simulink model "Control_car_position"  (R2022a)
settings: Solver=VariableStepAuto  StartTime=0.0  StopTime=100  RelTol=1e-3
libraries: slpidlib x5, simulink_extras x3
settings Model: Creator=jvlsq  LastModifiedBy=jvlsq
settings SolverCC: ZeroCrossAlgorithm=Adaptive
settings DebuggingCC: IgnoredZcDiagnostic=none

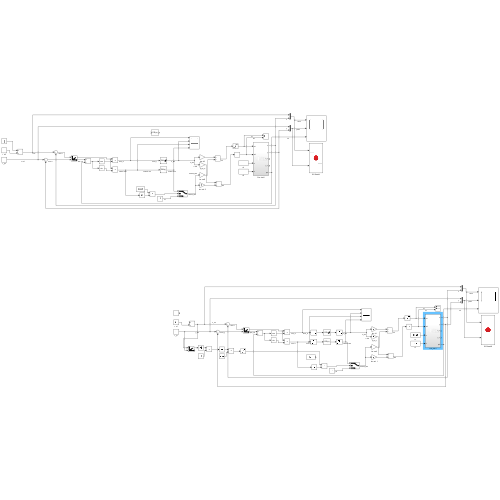
[thumbnail: Simulink's stored preview of the top-level diagram]
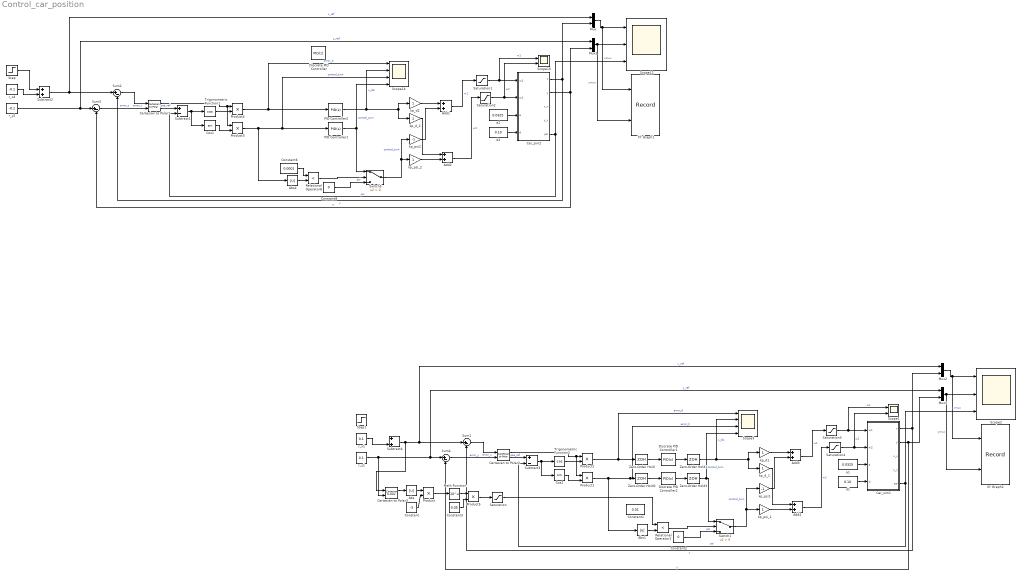
== system Control_car_position ==
  Abs : Abs  SaturateOnIntegerOverflow=off
  Abs1 : Abs  SaturateOnIntegerOverflow=off
  Abs4 : Abs  SaturateOnIntegerOverflow=off
  Add{1..4} (4 alike) : Sum
  Car_sim1 : Subsystem
  Car_sim2 : Subsystem
  Cartesian to Polar1 : simulink_extras/Transformations/Cartesian to Polar
  Cartesian to Polar2 : simulink_extras/Transformations/Cartesian to Polar
  Cartesian to Polar3 : simulink_extras/Transformations/Cartesian to Polar
  Constant : Constant  Value=-3
  Constant1 : Constant  Value=0.01
  Constant2 : Constant  Value=0
  Constant3 : Constant  Value=0.05
  Constant6 : Constant  Value=0.0001
  Constant8 : Constant  Value=0
  Cos1 : Trigonometry
  Cos2 : Trigonometry
  Discrete PID Controller : slpidlib/PID Controller  Controller=PID  Form=Parallel  TimeDomain=Discrete-time  UseExternalTs=off  SampleTime=-1  IntegratorMethod=Forward Euler  FilterMethod=Forward Euler  ControllerParametersSource=internal  P=1  I=1  UseKiTs=off  D=0  N=100  UseFilter=on  TunerSelectOption=Transfer Function Based (PID Tuner App)  InitialConditionSource=internal  InitialConditionForIntegrator=0  InitialConditionForFilter=0  DifferentiatorICPrevScaledInput=0  ExternalReset=none  TrackingMode=off  Kt=1  LimitOutput=off  SatLimitsSource=internal  UpperSaturationLimit=inf  LowerSaturationLimit=-inf  LinearizeAsGain=off  AntiWindupMode=none  Kb=1  POutMin=[]  POutMax=[]  IOutMin=[]  IOutMax=[]  DOutMin=[]  DOutMax=[]  NOutMin=[]  NOutMax=[]  SumOutMin=[]  SumOutMax=[]  SaturationOutMin=[]  SaturationOutMax=[]  PParamMin=[]  PParamMax=[]  IParamMin=[]  IParamMax=[]  DParamMin=[]  DParamMax=[]  NParamMin=[]  NParamMax=[]  KbParamMin=[]  KbParamMax=[]  KtParamMin=[]  KtParamMax=[]  KbOutMin=[]  KbOutMax=[]  KtOutMin=[]  KtOutMax=[]  IntegratorOutMin=[]  IntegratorOutMax=[]  FilterOutMin=[]  FilterOutMax=[]  SumI1OutMin=[]  SumI1OutMax=[]  SumI2OutMin=[]  SumI2OutMax=[]  SumI3OutMin=[]  SumI3OutMax=[]  SumI4OutMin=[]  SumI4OutMax=[]  SumDOutMin=[]  SumDOutMax=[]  DifferentiatorOutMin=[]  DifferentiatorOutMax=[]  FilterDiffOutCoefMin=[]  FilterDiffOutCoefMax=[]  ReciprocalOutMin=[]  ReciprocalOutMax=[]  SumDenOutMin=[]  SumDenOutMax=[]  SumNumOutMin=[]  SumNumOutMax=[]  DivideOutMin=[]  DivideOutMax=[]  UdiffTsProdOutMin=[]  UdiffTsProdOutMax=[]  NTsProdOutMin=[]  NTsProdOutMax=[]  UintegralTsProdOutMin=[]  UintegralTsProdOutMax=[]  UngainTsProdOutMin=[]  UngainTsProdOutMax=[]  IntegratorContinuousStateAttributes=''  IntegratorStateMustResolveToSignalObject=off  IntegratorRTWStateStorageClass=Auto  FilterContinuousStateAttributes=''  FilterStateMustResolveToSignalObject=off  FilterRTWStateStorageClass=Auto  ParallelPVariant=InternalParameters  IdealPVariant=Disabled  IVariant=InternalParameters  DVariant=InternalParameters  IntegratorVariant=Discrete  SatVariant=Disabled  AWVariant=Passthrough  PCopyVariant=Disabled  TRVariant=Disabled  FdbkBlocksVariant=Forward  IdealPFdbkVariant=Disabled  SatFdbkVariant=Disabled  DerivativeFilterVariant=ForwardEulerFilter  NVariant=InternalParameters  NCopyVariant=Disabled  FilterICVariant=InternalICsFilter  IntegratorICVariant=InternalICs  ExternalResetVariant=Disabled  TRSumVariant=Passthrough  SumFdbkVariant=Disabled  SumVariant=Sum_PID  TsampFilterVariant=InternalTs  TsampNgainVariant=Passthrough  TsampIntegralVariant=Passthrough  ExternalSaturationOutDataTypeStr=Inherit: Same as second input  aMode=0
  Discrete PID Controller1 : slpidlib/PID Controller  Controller=PID  Form=Parallel  TimeDomain=Discrete-time  UseExternalTs=off  SampleTime=-1  IntegratorMethod=Forward Euler  FilterMethod=Forward Euler  ControllerParametersSource=internal  P=30  I=1  UseKiTs=off  D=0  N=100  UseFilter=on  TunerSelectOption=Transfer Function Based (PID Tuner App)  InitialConditionSource=internal  InitialConditionForIntegrator=0  InitialConditionForFilter=0  DifferentiatorICPrevScaledInput=0  ExternalReset=none  TrackingMode=off  Kt=1  LimitOutput=on  SatLimitsSource=internal  UpperSaturationLimit=12  LowerSaturationLimit=-12  LinearizeAsGain=off  AntiWindupMode=clamping  Kb=1  POutMin=[]  POutMax=[]  IOutMin=[]  IOutMax=[]  DOutMin=[]  DOutMax=[]  NOutMin=[]  NOutMax=[]  SumOutMin=[]  SumOutMax=[]  SaturationOutMin=[]  SaturationOutMax=[]  PParamMin=[]  PParamMax=[]  IParamMin=[]  IParamMax=[]  DParamMin=[]  DParamMax=[]  NParamMin=[]  NParamMax=[]  KbParamMin=[]  KbParamMax=[]  KtParamMin=[]  KtParamMax=[]  KbOutMin=[]  KbOutMax=[]  KtOutMin=[]  KtOutMax=[]  IntegratorOutMin=[]  IntegratorOutMax=[]  FilterOutMin=[]  FilterOutMax=[]  SumI1OutMin=[]  SumI1OutMax=[]  SumI2OutMin=[]  SumI2OutMax=[]  SumI3OutMin=[]  SumI3OutMax=[]  SumI4OutMin=[]  SumI4OutMax=[]  SumDOutMin=[]  SumDOutMax=[]  DifferentiatorOutMin=[]  DifferentiatorOutMax=[]  FilterDiffOutCoefMin=[]  FilterDiffOutCoefMax=[]  ReciprocalOutMin=[]  ReciprocalOutMax=[]  SumDenOutMin=[]  SumDenOutMax=[]  SumNumOutMin=[]  SumNumOutMax=[]  DivideOutMin=[]  DivideOutMax=[]  UdiffTsProdOutMin=[]  UdiffTsProdOutMax=[]  NTsProdOutMin=[]  NTsProdOutMax=[]  UintegralTsProdOutMin=[]  UintegralTsProdOutMax=[]  UngainTsProdOutMin=[]  UngainTsProdOutMax=[]  IntegratorContinuousStateAttributes=''  IntegratorStateMustResolveToSignalObject=off  IntegratorRTWStateStorageClass=Auto  FilterContinuousStateAttributes=''  FilterStateMustResolveToSignalObject=off  FilterRTWStateStorageClass=Auto  ParallelPVariant=InternalParameters  IdealPVariant=Disabled  IVariant=InternalParameters  DVariant=InternalParameters  IntegratorVariant=Discrete  SatVariant=Enabled  AWVariant=DiscClampingParallel  PCopyVariant=Disabled  TRVariant=Disabled  FdbkBlocksVariant=Forward  IdealPFdbkVariant=Disabled  SatFdbkVariant=Disabled  DerivativeFilterVariant=ForwardEulerFilter  NVariant=InternalParameters  NCopyVariant=Disabled  FilterICVariant=InternalICsFilter  IntegratorICVariant=InternalICs  ExternalResetVariant=Disabled  TRSumVariant=Passthrough  SumFdbkVariant=Disabled  SumVariant=Sum_PID  TsampFilterVariant=InternalTs  TsampNgainVariant=Passthrough  TsampIntegralVariant=Passthrough  ExternalSaturationOutDataTypeStr=Inherit: Same as second input  aMode=0
  Discrete PID Controller2 : slpidlib/PID Controller  Controller=PID  Form=Parallel  TimeDomain=Discrete-time  UseExternalTs=off  SampleTime=-1  IntegratorMethod=Forward Euler  FilterMethod=Forward Euler  ControllerParametersSource=internal  P=100  I=0  UseKiTs=off  D=0  N=100  UseFilter=on  TunerSelectOption=Transfer Function Based (PID Tuner App)  InitialConditionSource=internal  InitialConditionForIntegrator=0  InitialConditionForFilter=0  DifferentiatorICPrevScaledInput=0  ExternalReset=none  TrackingMode=off  Kt=1  LimitOutput=off  SatLimitsSource=internal  UpperSaturationLimit=12  LowerSaturationLimit=0  LinearizeAsGain=off  AntiWindupMode=clamping  Kb=1  POutMin=[]  POutMax=[]  IOutMin=[]  IOutMax=[]  DOutMin=[]  DOutMax=[]  NOutMin=[]  NOutMax=[]  SumOutMin=[]  SumOutMax=[]  SaturationOutMin=[]  SaturationOutMax=[]  PParamMin=[]  PParamMax=[]  IParamMin=[]  IParamMax=[]  DParamMin=[]  DParamMax=[]  NParamMin=[]  NParamMax=[]  KbParamMin=[]  KbParamMax=[]  KtParamMin=[]  KtParamMax=[]  KbOutMin=[]  KbOutMax=[]  KtOutMin=[]  KtOutMax=[]  IntegratorOutMin=[]  IntegratorOutMax=[]  FilterOutMin=[]  FilterOutMax=[]  SumI1OutMin=[]  SumI1OutMax=[]  SumI2OutMin=[]  SumI2OutMax=[]  SumI3OutMin=[]  SumI3OutMax=[]  SumI4OutMin=[]  SumI4OutMax=[]  SumDOutMin=[]  SumDOutMax=[]  DifferentiatorOutMin=[]  DifferentiatorOutMax=[]  FilterDiffOutCoefMin=[]  FilterDiffOutCoefMax=[]  ReciprocalOutMin=[]  ReciprocalOutMax=[]  SumDenOutMin=[]  SumDenOutMax=[]  SumNumOutMin=[]  SumNumOutMax=[]  DivideOutMin=[]  DivideOutMax=[]  UdiffTsProdOutMin=[]  UdiffTsProdOutMax=[]  NTsProdOutMin=[]  NTsProdOutMax=[]  UintegralTsProdOutMin=[]  UintegralTsProdOutMax=[]  UngainTsProdOutMin=[]  UngainTsProdOutMax=[]  IntegratorContinuousStateAttributes=''  IntegratorStateMustResolveToSignalObject=off  IntegratorRTWStateStorageClass=Auto  FilterContinuousStateAttributes=''  FilterStateMustResolveToSignalObject=off  FilterRTWStateStorageClass=Auto  ParallelPVariant=InternalParameters  IdealPVariant=Disabled  IVariant=InternalParameters  DVariant=InternalParameters  IntegratorVariant=Discrete  SatVariant=Disabled  AWVariant=Passthrough  PCopyVariant=Disabled  TRVariant=Disabled  FdbkBlocksVariant=Forward  IdealPFdbkVariant=Disabled  SatFdbkVariant=Disabled  DerivativeFilterVariant=ForwardEulerFilter  NVariant=InternalParameters  NCopyVariant=Disabled  FilterICVariant=InternalICsFilter  IntegratorICVariant=InternalICs  ExternalResetVariant=Disabled  TRSumVariant=Passthrough  SumFdbkVariant=Disabled  SumVariant=Sum_PID  TsampFilterVariant=InternalTs  TsampNgainVariant=Passthrough  TsampIntegralVariant=Passthrough  ExternalSaturationOutDataTypeStr=Inherit: Same as second input  aMode=0
  Math Function : Math  Operator=10^u
  Mux{,1..3} (4 alike) : Mux  Inputs=2
  PID Controller1 : slpidlib/PID Controller  Controller=PID  Form=Parallel  TimeDomain=Continuous-time  UseExternalTs=off  SampleTime=-1  IntegratorMethod=Forward Euler  FilterMethod=Forward Euler  ControllerParametersSource=internal  P=100  I=0  UseKiTs=off  D=0  N=100  UseFilter=on  TunerSelectOption=Transfer Function Based (PID Tuner App)  InitialConditionSource=internal  InitialConditionForIntegrator=0  InitialConditionForFilter=0  DifferentiatorICPrevScaledInput=0  ExternalReset=none  TrackingMode=off  Kt=1  LimitOutput=off  SatLimitsSource=internal  UpperSaturationLimit=inf  LowerSaturationLimit=-inf  LinearizeAsGain=on  AntiWindupMode=none  Kb=1  POutMin=[]  POutMax=[]  IOutMin=[]  IOutMax=[]  DOutMin=[]  DOutMax=[]  NOutMin=[]  NOutMax=[]  SumOutMin=[]  SumOutMax=[]  SaturationOutMin=[]  SaturationOutMax=[]  PParamMin=[]  PParamMax=[]  IParamMin=[]  IParamMax=[]  DParamMin=[]  DParamMax=[]  NParamMin=[]  NParamMax=[]  KbParamMin=[]  KbParamMax=[]  KtParamMin=[]  KtParamMax=[]  KbOutMin=[]  KbOutMax=[]  KtOutMin=[]  KtOutMax=[]  IntegratorOutMin=[]  IntegratorOutMax=[]  FilterOutMin=[]  FilterOutMax=[]  SumI1OutMin=[]  SumI1OutMax=[]  SumI2OutMin=[]  SumI2OutMax=[]  SumI3OutMin=[]  SumI3OutMax=[]  SumI4OutMin=[]  SumI4OutMax=[]  SumDOutMin=[]  SumDOutMax=[]  DifferentiatorOutMin=[]  DifferentiatorOutMax=[]  FilterDiffOutCoefMin=[]  FilterDiffOutCoefMax=[]  ReciprocalOutMin=[]  ReciprocalOutMax=[]  SumDenOutMin=[]  SumDenOutMax=[]  SumNumOutMin=[]  SumNumOutMax=[]  DivideOutMin=[]  DivideOutMax=[]  UdiffTsProdOutMin=[]  UdiffTsProdOutMax=[]  NTsProdOutMin=[]  NTsProdOutMax=[]  UintegralTsProdOutMin=[]  UintegralTsProdOutMax=[]  UngainTsProdOutMin=[]  UngainTsProdOutMax=[]  IntegratorContinuousStateAttributes=''  IntegratorStateMustResolveToSignalObject=off  IntegratorRTWStateStorageClass=Auto  FilterContinuousStateAttributes=''  FilterStateMustResolveToSignalObject=off  FilterRTWStateStorageClass=Auto  ParallelPVariant=InternalParameters  IdealPVariant=Disabled  IVariant=InternalParameters  DVariant=InternalParameters  IntegratorVariant=Continuous  SatVariant=Disabled  AWVariant=Passthrough  PCopyVariant=Disabled  TRVariant=Disabled  FdbkBlocksVariant=Forward  IdealPFdbkVariant=Disabled  SatFdbkVariant=Disabled  DerivativeFilterVariant=ContFilter  NVariant=InternalParameters  NCopyVariant=Disabled  FilterICVariant=InternalICsFilter  IntegratorICVariant=InternalICs  ExternalResetVariant=Disabled  TRSumVariant=Passthrough  SumFdbkVariant=Disabled  SumVariant=Sum_PID  TsampFilterVariant=InternalTs  TsampNgainVariant=Passthrough  TsampIntegralVariant=Passthrough  ExternalSaturationOutDataTypeStr=Inherit: Same as second input  aMode=0
  PID Controller2 : slpidlib/PID Controller  Controller=PID  Form=Parallel  TimeDomain=Continuous-time  UseExternalTs=off  SampleTime=-1  IntegratorMethod=Forward Euler  FilterMethod=Forward Euler  ControllerParametersSource=internal  P=30  I=1  UseKiTs=off  D=0  N=100  UseFilter=on  TunerSelectOption=Transfer Function Based (PID Tuner App)  InitialConditionSource=internal  InitialConditionForIntegrator=0  InitialConditionForFilter=0  DifferentiatorICPrevScaledInput=0  ExternalReset=none  TrackingMode=off  Kt=1  LimitOutput=on  SatLimitsSource=internal  UpperSaturationLimit=12  LowerSaturationLimit=-12  LinearizeAsGain=on  AntiWindupMode=clamping  Kb=1  POutMin=[]  POutMax=[]  IOutMin=[]  IOutMax=[]  DOutMin=[]  DOutMax=[]  NOutMin=[]  NOutMax=[]  SumOutMin=[]  SumOutMax=[]  SaturationOutMin=[]  SaturationOutMax=[]  PParamMin=[]  PParamMax=[]  IParamMin=[]  IParamMax=[]  DParamMin=[]  DParamMax=[]  NParamMin=[]  NParamMax=[]  KbParamMin=[]  KbParamMax=[]  KtParamMin=[]  KtParamMax=[]  KbOutMin=[]  KbOutMax=[]  KtOutMin=[]  KtOutMax=[]  IntegratorOutMin=[]  IntegratorOutMax=[]  FilterOutMin=[]  FilterOutMax=[]  SumI1OutMin=[]  SumI1OutMax=[]  SumI2OutMin=[]  SumI2OutMax=[]  SumI3OutMin=[]  SumI3OutMax=[]  SumI4OutMin=[]  SumI4OutMax=[]  SumDOutMin=[]  SumDOutMax=[]  DifferentiatorOutMin=[]  DifferentiatorOutMax=[]  FilterDiffOutCoefMin=[]  FilterDiffOutCoefMax=[]  ReciprocalOutMin=[]  ReciprocalOutMax=[]  SumDenOutMin=[]  SumDenOutMax=[]  SumNumOutMin=[]  SumNumOutMax=[]  DivideOutMin=[]  DivideOutMax=[]  UdiffTsProdOutMin=[]  UdiffTsProdOutMax=[]  NTsProdOutMin=[]  NTsProdOutMax=[]  UintegralTsProdOutMin=[]  UintegralTsProdOutMax=[]  UngainTsProdOutMin=[]  UngainTsProdOutMax=[]  IntegratorContinuousStateAttributes=''  IntegratorStateMustResolveToSignalObject=off  IntegratorRTWStateStorageClass=Auto  FilterContinuousStateAttributes=''  FilterStateMustResolveToSignalObject=off  FilterRTWStateStorageClass=Auto  ParallelPVariant=InternalParameters  IdealPVariant=Disabled  IVariant=InternalParameters  DVariant=InternalParameters  IntegratorVariant=Continuous  SatVariant=Enabled  AWVariant=ContClampingParallel  PCopyVariant=Disabled  TRVariant=Disabled  FdbkBlocksVariant=Forward  IdealPFdbkVariant=Disabled  SatFdbkVariant=Disabled  DerivativeFilterVariant=ContFilter  NVariant=InternalParameters  NCopyVariant=Disabled  FilterICVariant=InternalICsFilter  IntegratorICVariant=InternalICs  ExternalResetVariant=Disabled  TRSumVariant=Passthrough  SumFdbkVariant=Disabled  SumVariant=Sum_PID  TsampFilterVariant=InternalTs  TsampNgainVariant=Passthrough  TsampIntegralVariant=Passthrough  ExternalSaturationOutDataTypeStr=Inherit: Same as second input  aMode=0
  Product{,1..5} (6 alike) : Product
  Relational Operator1 : RelationalOperator  Operator=<  OutDataTypeStr=boolean  RndMeth=Simplest  InputSameDT=off
  Relational Operator8 : RelationalOperator  Operator=<  OutDataTypeStr=boolean  RndMeth=Simplest  InputSameDT=off
  Saturation : Saturate  UpperLimit=0.01  LowerLimit=0.0001
  Saturation{1..4} (4 alike) : Saturate  UpperLimit=12  LowerLimit=-12
  Scope1 : Scope  NumInputPorts=2
  Scope10 : Scope  NumInputPorts=2
  Scope12 : Scope  NumInputPorts=3
  Scope14 : Scope  NumInputPorts=4
  Scope2 : Scope  NumInputPorts=3
  Scope3 : Scope  NumInputPorts=4
  Step : Step  Time=7  After=0.5  SampleTime=0
  Step1 : Step  Time=7  After=2  SampleTime=0
  Subtract1 : Sum  Inputs=+-
  Subtract2 : Sum
  Subtract3 : Sum  Inputs=+-
  Subtract4 : Sum
  Sum{1..4} (4 alike) : Sum  Inputs=|+-
  Switch1 : Switch  Criteria=u2 > Threshold  SaturateOnIntegerOverflow=off  InputSameDT=off
  Switch5 : Switch  Criteria=u2 > Threshold  SaturateOnIntegerOverflow=off  InputSameDT=off
  Trigonometric Function1 : Trigonometry  Operator=cos
  Trigonometric Function2 : Trigonometry  Operator=cos
  XY Graph1 : Record  FileSettingsInternal="{\"entries\":[{\"content\":{\"excelSettings\":{\"content\":{},\"type\":\"Streamout.ExcelSettings\"}},\"type\":\"Streamout.FileSettingStorage\",\"uuid\":\"d923e3af-334a-4ac6-94b0-767c2d3f18a5\"}],\"packageUris\":[\"http://schema.mathworks.com/mf0/streamout_blocks/R2020a\"],\"version\":\"1.0\"}"  Layout=[1 1]  SignalsInternal="{\"entries\":[{\"content\":{\"signals\":[{\"content\":{\"blockPath\":[\"Control_car_position/XY Graph1\"],\"channel\":[],\"dimensions\":[2],\"domain\":\"Control_car_position/XY Graph1\",\"hasChildren\":true,\"lineColor\":\"#0072bd\",\"plots\":[],\"port\":1,\"sid\":[\"\"],\"signalID\":856,\"signalName\":\"xmux\"},\"type\":\"RecordBlkView.Signal\",\"uuid\":\"d70a9752-5393-4ad4-a36b-ddbcda4d9cba\"},{\"content\":{\"blockPath\":[\"Control_car_position/XY Graph1\"],\"channel\":[1],\"dimensions\":[2],\"domain\":\"Control_car_position/XY Graph1\",\"lineColor\":\"#fe330a\",\"lineStyle\":\"DASH_DOT\",\"parentID\":856,\"plots\":[1],\"port\":1,\"sid\":[\"\"],\"signalID\":857,\"signalName\":\"xmux\"},\"type\":\"RecordBlkView.Signal\",\"uuid\":\"8dfb860c-e4e5-4e22-82b4-c9c49d44ed48\"},{\"content\":{\"blockPath\":[\"Control_car_position/XY Graph1\"],\"channel\":[],\"dimensions\":[2],\"domain\":\"Control_car_position/XY Graph1\",\"hasChildren\":true,\"lineColor\":\"#edb120\",\"plots\":[],\"port\":2,\"sid\":[\"\"],\"signalID\":861,\"signalName\":\"ymux\"},\"type\":\"RecordBlkView.Signal\",\"uuid\":\"5bae06c2-901e-4742-97f1-c8c1ff39c41a\"},{\"content\":{\"blockPath\":[\"Control_car_position/XY Graph1\"],\"channel\":[1],\"dimensions\":[2],\"domain\":\"Control_car_position/XY Graph1\",\"lineColor\":\"#4dbeee\",\"lineStyle\":\"DASHED\",\"parentID\":861,\"plots\":[1],\"port\":2,\"sid\":[\"\"],\"signalID\":862,\"signalName\":\"ymux\"},\"type\":\"RecordBlkView.Signal\",\"uuid\":\"5bfa4c18-6904-4296-a2d5-2c5913434ad1\"},{\"content\":{\"blockPath\":[\"Control_car_position/XY Graph1\"],\"channel\":[2],\"dimensions\":[2],\"domain\":\"Control_car_position/XY Graph1\",\"lineColor\":\"#fe330a\",\"lineStyle\":\"DASH_DOT\",\"parentID\":856,\"plots\":[1],\"port\":1,\"sid\":[\"\"],\"signalID\":868,\"signalName\":\"xmux\"},\"type\":\"RecordBlkView.Signal\",\"uuid\":\"065bae5f-0713-48a9-8290-736caceba6c6\"},{\"content\":{\"blockPath\":[\"Control_car_position/XY Graph1\"],\"channel\":[2],\"dimensions\":[2],\"domain\":\"Control_car_position/XY Graph1\",\"lineColor\":\"#139fff\",\"lineStyle\":\"DASHED\",\"parentID\":861,\"plots\":[1],\"port\":2,\"sid\":[\"\"],\"signalID\":869,\"signalName\":\"ymux\"},\"type\":\"RecordBlkView.Signal\",\"uuid\":\"5299f899-2536-473b-be2d-5ad89941e321\"}]},\"type\":\"RecordBlkView.InputSignals\",\"uuid\":\"c07bf6ee-6508-4234-8602-a6eebd21dbd2\"}],\"packageUris\":[\"http://schema.mathworks.com/mf0/streamout_blocks/R2020a\"],\"version\":\"1.0\"}"  VisualizationBindings="{\"xyplotplugin\":{\"info\":[{\"series\":[{\"bindingParametersList\":[{\"parameter\":\"X-Axis\",\"signalID\":868,\"signalName\":\"xmux(2)\"},{\"parameter\":\"Y-Axis\",\"signalID\":869,\"signalName\":\"ymux(2)\"}],\"seriesID\":39394},{\"bindingParametersList\":[{\"parameter\":\"X-Axis\",\"signalID\":857,\"signalName\":\"xmux(1)\"},{\"parameter\":\"Y-Axis\",\"signalID\":862,\"signalName\":\"ymux(1)\"}],\"seriesID\":35653}],\"subplotID\":1}]}}"  CompatibilityTag=XY
  XY Graph2 : Record  FileSettingsInternal="{\"entries\":[{\"content\":{\"excelSettings\":{\"content\":{},\"type\":\"Streamout.ExcelSettings\"}},\"type\":\"Streamout.FileSettingStorage\",\"uuid\":\"932c3877-a841-4e40-bfb4-26097e341148\"}],\"packageUris\":[\"http://schema.mathworks.com/mf0/streamout_blocks/R2020a\"],\"version\":\"1.0\"}"  Layout=[1 1]  SignalsInternal="{\"entries\":[{\"content\":{\"signals\":[{\"content\":{\"blockPath\":[\"Control_car_position/XY Graph2\"],\"channel\":[],\"dimensions\":[2],\"domain\":\"Control_car_position/XY Graph2\",\"hasChildren\":true,\"lineColor\":\"#64d413\",\"plots\":[],\"port\":1,\"sid\":[\"\"],\"signalID\":846,\"signalName\":\"xmux\"},\"type\":\"RecordBlkView.Signal\",\"uuid\":\"3d4edf9f-2018-47c3-be2b-6121539d543f\"},{\"content\":{\"blockPath\":[\"Control_car_position/XY Graph2\"],\"channel\":[1],\"dimensions\":[2],\"domain\":\"Control_car_position/XY Graph2\",\"lineColor\":\"#22b573\",\"parentID\":846,\"plots\":[1],\"port\":1,\"sid\":[\"\"],\"signalID\":847,\"signalName\":\"xmux\"},\"type\":\"RecordBlkView.Signal\",\"uuid\":\"a9140721-4141-45ae-82c9-b33303add108\"},{\"content\":{\"blockPath\":[\"Control_car_position/XY Graph2\"],\"channel\":[],\"dimensions\":[2],\"domain\":\"Control_car_position/XY Graph2\",\"hasChildren\":true,\"lineColor\":\"#fe330a\",\"plots\":[],\"port\":2,\"sid\":[\"\"],\"signalID\":851,\"signalName\":\"ymux\"},\"type\":\"RecordBlkView.Signal\",\"uuid\":\"16ea9268-7951-4b05-9a0d-a992f5a2a733\"},{\"content\":{\"blockPath\":[\"Control_car_position/XY Graph2\"],\"channel\":[1],\"dimensions\":[2],\"domain\":\"Control_car_position/XY Graph2\",\"lineColor\":\"#d95319\",\"parentID\":851,\"plots\":[1],\"port\":2,\"sid\":[\"\"],\"signalID\":852,\"signalName\":\"ymux\"},\"type\":\"RecordBlkView.Signal\",\"uuid\":\"ff227041-aef3-46e5-b684-eeeff846abd3\"},{\"content\":{\"blockPath\":[\"Control_car_position/XY Graph2\"],\"channel\":[2],\"dimensions\":[2],\"domain\":\"Control_car_position/XY Graph2\",\"lineColor\":\"#a2142f\",\"parentID\":846,\"plots\":[1],\"port\":1,\"sid\":[\"\"],\"signalID\":866,\"signalName\":\"xmux\"},\"type\":\"RecordBlkView.Signal\",\"uuid\":\"f856e686-e868-4650-859d-0ed1042a01ca\"},{\"content\":{\"blockPath\":[\"Control_car_position/XY Graph2\"],\"channel\":[2],\"dimensions\":[2],\"domain\":\"Control_car_position/XY Graph2\",\"lineColor\":\"#139fff\",\"parentID\":851,\"plots\":[1],\"port\":2,\"sid\":[\"\"],\"signalID\":867,\"signalName\":\"ymux\"},\"type\":\"RecordBlkView.Signal\",\"uuid\":\"81383463-0dfd-47f0-9c5b-b8cf9b4f73a8\"}]},\"type\":\"RecordBlkView.InputSignals\",\"uuid\":\"e31c9e6a-c858-4e64-b58d-d3c5244947a3\"}],\"packageUris\":[\"http://schema.mathworks.com/mf0/streamout_blocks/R2020a\"],\"version\":\"1.0\"}"  VisualizationBindings="{\"xyplotplugin\":{\"info\":[{\"series\":[{\"bindingParametersList\":[{\"parameter\":\"X-Axis\",\"signalID\":847,\"signalName\":\"xmux(1)\"},{\"parameter\":\"Y-Axis\",\"signalID\":852,\"signalName\":\"ymux(1)\"}],\"seriesID\":23175},{\"bindingParametersList\":[{\"parameter\":\"X-Axis\",\"signalID\":866,\"signalName\":\"xmux(2)\"},{\"parameter\":\"Y-Axis\",\"signalID\":867,\"signalName\":\"ymux(2)\"}],\"seriesID\":57963}],\"subplotID\":1}]}}"  CompatibilityTag=XY
  Zero-Order Hold{,1..3} (4 alike) : ZeroOrderHold  SampleTime=0.016
  a1 : Constant  Value=0.0325
  a2 : Constant  Value=0.0325
  d1 : Constant  Value=0.10
  d2 : Constant  Value=0.10
  kp_d1 : Gain
  kp_d2 : Gain
  kp_d_1 : Gain
  kp_d_2 : Gain
  kp_psi1 : Gain  Gain=-1
  kp_psi2 : Gain  Gain=-1
  kp_psi_1 : Gain
  kp_psi_2 : Gain
  r_x1 : Constant  Value=0.1
  r_x4 : Constant  Value=-0.1
  r_y1 : Constant  Value=0.1
  r_y2 : Constant  Value=-0.1
  wires:
  Cartesian to Polar1/1 -> Product4/1, Product3/1
  Cartesian to Polar1/2 -> Subtract1/1  "pse_ref"
  Product4/1 -> PID Controller2/1, Scope14/1  "error_d"
  Cos1/1 -> Product3/2
  Subtract1/1 -> Cos1/1, Trigonometric Function1/1
  r_x4/1 -> Subtract2/2
  Saturation2/1 -> Car_sim2/2(w2), Scope10/2  "w2"
  d2/1 -> Car_sim2/4(d)
  Add2/1 -> Saturation2/1  "w2"
  PID Controller2/1 -> Scope14/2, kp_d_2/1, kp_d2/1  "u_dis"
  Sum2/1 -> Cartesian to Polar1/1  "error_x"
  Car_sim2/1(x) -> Mux/2, Sum2/2  "x"
  Car_sim2/2(y) -> Mux1/2, Sum3/2  "y"
  Sum3/1 -> Cartesian to Polar1/2  "error_y"
  Saturation1/1 -> Car_sim2/1(w1), Scope10/1  "w1"
  Car_sim2/5(psi) -> Scope12/3, Subtract1/2  "psi"
  Switch5/1 -> kp_psi2/1, kp_psi_2/1  "control_turn"
  kp_d2/1 -> Add1/1
  kp_psi2/1 -> Add1/2
  Add1/1 -> Saturation1/1  "w1"
  r_y2/1 -> Mux1/1, Sum3/1  "y_ref"
  a2/1 -> Car_sim2/3(a)
  kp_d_2/1 -> Add2/1
  kp_psi_2/1 -> Add2/2
  Trigonometric Function1/1 -> Product4/2
  PID Controller1/1 -> Switch5/1, Scope14/4  "control_turn"
  Subtract2/1 -> Sum2/1, Mux/1  "x_ref"
  Step/1 -> Subtract2/1
  Mux/1 -> XY Graph1/1, Scope12/1  "xmux"
  Mux1/1 -> XY Graph1/2, Scope12/2  "ymux"
  Abs4/1 -> Relational Operator8/2
  Constant6/1 -> Relational Operator8/1
  Relational Operator8/1 -> Switch5/2
  Constant8/1 -> Switch5/3  "psi"
  Product3/1 -> Abs4/1, PID Controller1/1, Scope14/3  "control_turn"
  Product1/1 -> Abs1/1, Scope3/3, Zero-Order Hold2/1  "error_h"
  Subtract4/1 -> Cartesian to Polar3/1, Sum1/1, Mux2/1  "x_ref"
  kp_psi_1/1 -> Add4/2
  kp_psi1/1 -> Add3/2
  Add3/1 -> Saturation3/1  "w1"
  r_y1/1 -> Cartesian to Polar3/2, Mux3/1, Sum4/1  "y_ref"
  Saturation3/1 -> Car_sim1/1(w1), Scope1/1  "w1"
  Car_sim1/2(y) -> Mux3/2, Sum4/2  "y"
  Sum4/1 -> Cartesian to Polar2/2  "error_y"
  Sum1/1 -> Cartesian to Polar2/1  "error_x"
  Zero-Order Hold1/1 -> Scope3/2, kp_d_1/1, kp_d1/1  "u_dis"
  Add4/1 -> Saturation4/1  "w2"
  Constant2/1 -> Switch1/3  "psi"
  r_x1/1 -> Subtract4/2
  Cos2/1 -> Product1/2
  kp_d_1/1 -> Add4/1
  Product2/1 -> Zero-Order Hold/1, Scope3/1  "error_d"
  Cartesian to Polar2/1 -> Product2/1, Product1/1
  Cartesian to Polar2/2 -> Subtract3/1  "pse_ref"
  Subtract3/1 -> Cos2/1, Trigonometric Function2/1
  Mux3/1 -> XY Graph2/2, Scope2/2  "ymux"
  Zero-Order Hold3/1 -> Switch1/1, Scope3/4  "control_turn"
  Car_sim1/1(x) -> Mux2/2, Sum1/2  "x"
  Mux2/1 -> XY Graph2/1, Scope2/1  "xmux"
  Trigonometric Function2/1 -> Product2/2
  Abs1/1 -> Relational Operator1/2
  d1/1 -> Car_sim1/4(d)
  Car_sim1/5(psi) -> Scope2/3, Subtract3/2  "psi"
  a1/1 -> Car_sim1/3(a)
  Saturation4/1 -> Car_sim1/2(w2), Scope1/2  "w2"
  kp_d1/1 -> Add3/1
  Relational Operator1/1 -> Switch1/2
  Zero-Order Hold/1 -> Discrete PID Controller1/1
  Discrete PID Controller1/1 -> Zero-Order Hold1/1
  Discrete PID Controller2/1 -> Zero-Order Hold3/1
  Zero-Order Hold2/1 -> Discrete PID Controller2/1
  Cartesian to Polar3/1 -> Abs/1
  Abs/1 -> Product/1
  Constant/1 -> Product/2
  Product/1 -> Math Function/1
  Math Function/1 -> Product5/1
  Constant3/1 -> Product5/2
  Product5/1 -> Saturation/1
  Saturation/1 -> Relational Operator1/1
  Switch1/1 -> kp_psi_1/1, kp_psi1/1  "control_turn"

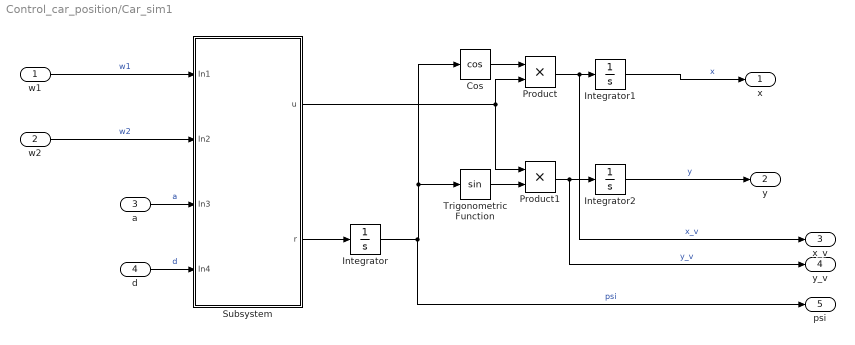
== system Control_car_position/Car_sim1 ==
  w1 : Inport
  w2 : Inport  Port=2
  a : Inport  Port=3
  d : Inport  Port=4
  Cos : Trigonometry  Operator=cos
  Integrator : Integrator
  Integrator1 : Integrator
  Integrator2 : Integrator
  Product : Product
  Product1 : Product
  Subsystem : Subsystem
  Trigonometric Function : Trigonometry
  x : Outport
  y : Outport  Port=2
  x_v : Outport  Port=3
  y_v : Outport  Port=4
  psi : Outport  Port=5
  wires:
  Product1/1 -> y_v/1, Integrator2/1  "y_v"
  Integrator1/1 -> x/1  "x"
  Integrator/1 -> psi/1, Trigonometric Function/1, Cos/1  "psi"
  Subsystem/1(u) -> Product/2, Product1/1
  Trigonometric Function/1 -> Product1/2
  d/1 -> Subsystem/4(In4)  "d"
  Product/1 -> x_v/1, Integrator1/1  "x_v"
  Subsystem/2(r) -> Integrator/1
  Cos/1 -> Product/1
  a/1 -> Subsystem/3(In3)  "a"
  Integrator2/1 -> y/1  "y"
  w1/1 -> Subsystem/1(In1)  "w1"
  w2/1 -> Subsystem/2(In2)  "w2"

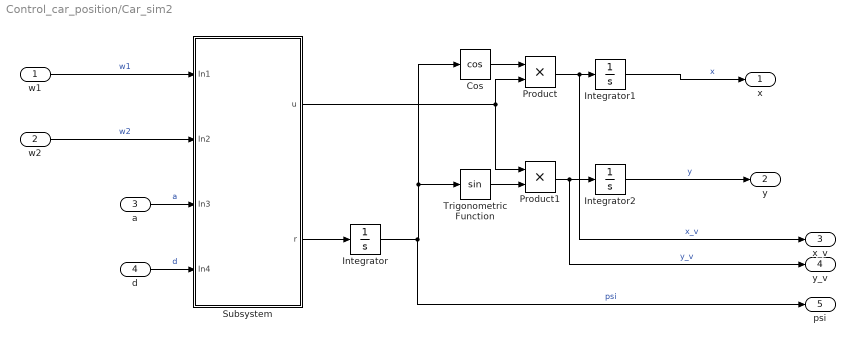
== system Control_car_position/Car_sim2 ==
  w1 : Inport
  w2 : Inport  Port=2
  a : Inport  Port=3
  d : Inport  Port=4
  Cos : Trigonometry  Operator=cos
  Integrator : Integrator
  Integrator1 : Integrator
  Integrator2 : Integrator
  Product : Product
  Product1 : Product
  Subsystem : Subsystem
  Trigonometric Function : Trigonometry
  x : Outport
  y : Outport  Port=2
  x_v : Outport  Port=3
  y_v : Outport  Port=4
  psi : Outport  Port=5
  wires:
  Product1/1 -> y_v/1, Integrator2/1  "y_v"
  Integrator1/1 -> x/1  "x"
  Integrator/1 -> psi/1, Trigonometric Function/1, Cos/1  "psi"
  Subsystem/1(u) -> Product/2, Product1/1
  Trigonometric Function/1 -> Product1/2
  d/1 -> Subsystem/4(In4)  "d"
  Product/1 -> x_v/1, Integrator1/1  "x_v"
  Subsystem/2(r) -> Integrator/1
  Cos/1 -> Product/1
  a/1 -> Subsystem/3(In3)  "a"
  Integrator2/1 -> y/1  "y"
  w1/1 -> Subsystem/1(In1)  "w1"
  w2/1 -> Subsystem/2(In2)  "w2"

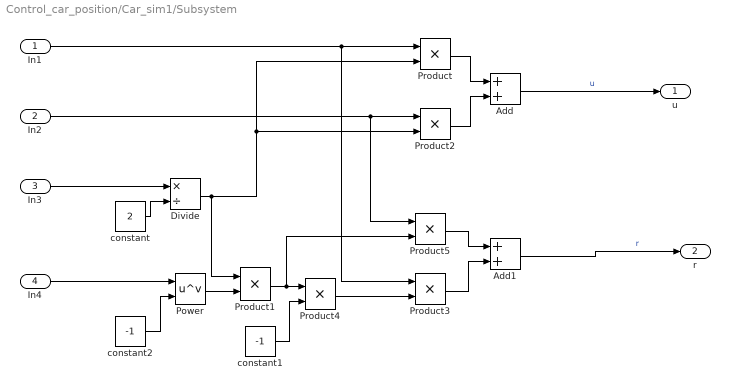
== system Control_car_position/Car_sim1/Subsystem ==
  In1 : Inport
  In2 : Inport  Port=2
  In3 : Inport  Port=3
  In4 : Inport  Port=4
  Add : Sum
  Add1 : Sum
  Divide : Product  Inputs=*/
  Power : Math  Operator=pow
  Product{,1..5} (6 alike) : Product
  constant : Constant  Value=2
  constant1 : Constant  Value=-1
  constant2 : Constant  Value=-1
  u : Outport
  r : Outport  Port=2
  wires:
  constant1/1 -> Product4/2
  In2/1 -> Product5/1, Product2/1
  Divide/1 -> Product2/2, Product/2, Product1/1
  Product3/1 -> Add1/2
  Product1/1 -> Product5/2, Product4/1
  In4/1 -> Power/1
  constant2/1 -> Power/2
  In1/1 -> Product3/1, Product/1
  Product2/1 -> Add/2
  Product5/1 -> Add1/1
  Product4/1 -> Product3/2
  constant/1 -> Divide/2
  Add/1 -> u/1  "u"
  Add1/1 -> r/1  "r"
  Product/1 -> Add/1
  Power/1 -> Product1/2
  In3/1 -> Divide/1

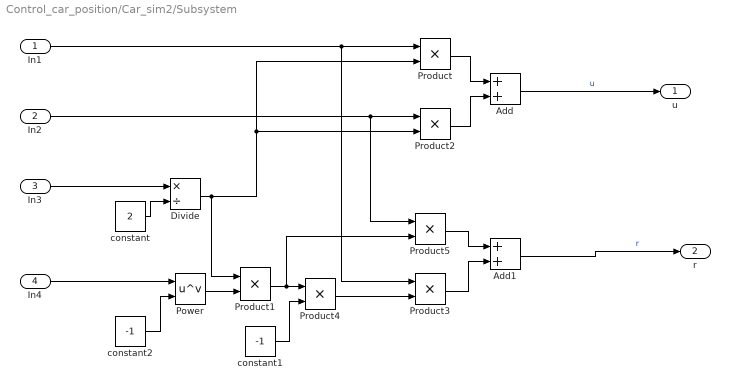
== system Control_car_position/Car_sim2/Subsystem ==
  In1 : Inport
  In2 : Inport  Port=2
  In3 : Inport  Port=3
  In4 : Inport  Port=4
  Add : Sum
  Add1 : Sum
  Divide : Product  Inputs=*/
  Power : Math  Operator=pow
  Product{,1..5} (6 alike) : Product
  constant : Constant  Value=2
  constant1 : Constant  Value=-1
  constant2 : Constant  Value=-1
  u : Outport
  r : Outport  Port=2
  wires:
  constant1/1 -> Product4/2
  In2/1 -> Product5/1, Product2/1
  Divide/1 -> Product2/2, Product/2, Product1/1
  Product3/1 -> Add1/2
  Product1/1 -> Product5/2, Product4/1
  In4/1 -> Power/1
  constant2/1 -> Power/2
  In1/1 -> Product3/1, Product/1
  Product2/1 -> Add/2
  Product5/1 -> Add1/1
  Product4/1 -> Product3/2
  constant/1 -> Divide/2
  Add/1 -> u/1  "u"
  Add1/1 -> r/1  "r"
  Product/1 -> Add/1
  Power/1 -> Product1/2
  In3/1 -> Divide/1
